simulink model "backup"  (R2015b)
settings: Solver=VariableStepAuto  StartTime=0.0  StopTime=10.0  RelTol=1e-3
undefined symbols (not defined in the file or in its folder): ad, aq, bd, bq, cd, cq, n1, T
settings Model: Creator=Martin Andersen  LastModifiedBy=Martin Andersen

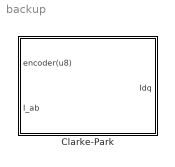
== system backup ==
  Clarke-Park : Subsystem  SystemSampleTime=T

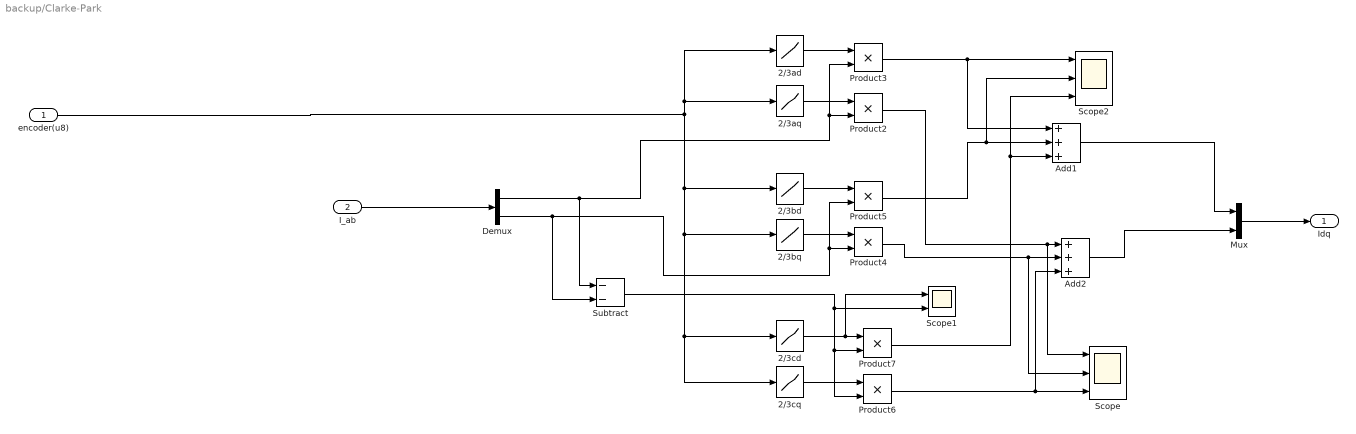
== system backup/Clarke-Park ==
  encoder(u8) : Inport
  I_ab : Inport  Port=2
  2/3ad : Lookup_n-D  NumberOfTableDimensions=1  BreakpointsForDimension1=n1  Table=ad*2/3  InterpMethod=Nearest  InternalRulePriority=Speed  RndMeth=Simplest  InputSameDT=on
  2/3aq : Lookup_n-D  NumberOfTableDimensions=1  BreakpointsForDimension1=n1  Table=aq*2/3  InterpMethod=Nearest  InternalRulePriority=Speed  RndMeth=Simplest  InputSameDT=on
  2/3bd : Lookup_n-D  NumberOfTableDimensions=1  BreakpointsForDimension1=n1  Table=bd*2/3  InterpMethod=Nearest  InternalRulePriority=Speed  RndMeth=Simplest  InputSameDT=on
  2/3bq : Lookup_n-D  NumberOfTableDimensions=1  BreakpointsForDimension1=n1  Table=bq*2/3  InterpMethod=Nearest  InternalRulePriority=Speed  RndMeth=Simplest  InputSameDT=on
  2/3cd : Lookup_n-D  NumberOfTableDimensions=1  BreakpointsForDimension1=n1  Table=cd*2/3  InterpMethod=Nearest  InternalRulePriority=Speed  RndMeth=Simplest  InputSameDT=on
  2/3cq : Lookup_n-D  NumberOfTableDimensions=1  BreakpointsForDimension1=n1  Table=cq*2/3  InterpMethod=Nearest  InternalRulePriority=Speed  RndMeth=Simplest  InputSameDT=on
  Add1 : Sum  Inputs=+++
  Add2 : Sum  Inputs=+++
  Demux : Demux  Outputs=2
  Mux : Mux  Inputs=2
  Product{2..7} (6 alike) : Product
  Scope : Scope  NumInputPorts=3
  Scope1 : Scope  NumInputPorts=2
  Scope2 : Scope  NumInputPorts=3
  Subtract : Sum  Inputs=--
  Idq : Outport
  wires:
  Add2/1 -> Mux/2
  2/3ad/1 -> Product3/1
  2/3cq/1 -> Product6/1
  Demux/1 -> Product2/2, Product3/2, Subtract/1
  2/3bq/1 -> Product4/1
  I_ab/1 -> Demux/1
  Subtract/1 -> Product6/2, Product7/2, Scope1/2
  Product6/1 -> Scope/3, Add2/3
  Product4/1 -> Scope/2, Add2/2
  2/3aq/1 -> Product2/1
  Product5/1 -> Scope2/2, Add1/2
  2/3bd/1 -> Product5/1
  Demux/2 -> Subtract/2, Product5/2, Product4/2
  2/3cd/1 -> Scope1/1, Product7/1
  Product3/1 -> Scope2/1, Add1/1
  Product2/1 -> Scope/1, Add2/1
  Product7/1 -> Scope2/3, Add1/3
  encoder(u8)/1 -> 2/3cq/1, 2/3cd/1, 2/3bq/1, 2/3bd/1, 2/3aq/1, 2/3ad/1
  Mux/1 -> Idq/1
  Add1/1 -> Mux/1
